simulink library "library_mtu_simulink"  (R2018a)
settings: Solver=VariableStepAuto  StartTime=0.0  StopTime=10.0  RelTol=1e-3  EnableMultiTasking=on
undefined symbols (not defined in the file or in its folder): AP, MP, PA
settings Model: Creator=danielhaeufle  LastModifiedBy=katrinstollenmaier
settings DataIOCC: LimitDataPoints=on
settings OptimizationCC: LifeSpan=inf
settings DebuggingCC: AllowSymbolicDim=off  SFUnexpectedBacktrackingDiag=warning  SFNoUnconditionalDefaultTransitionDiag=warning  SFExecutionAtInitializationDiag=none
settings ModelReferenceCC: PropagateSignalLabelsOutOfModel=off
settings CodeAppCC: StateflowObjectComments=on
settings GRTTargetCC: TargetLangStandard=C89/C90 (ANSI)
settings ConfigComp: CovMetricSettings=dw  CovHtmlReporting=on  CovSaveCumulativeToWorkspaceVar=on  CovSaveSingleToWorkspaceVar=on  CovExternalEMLEnable=off

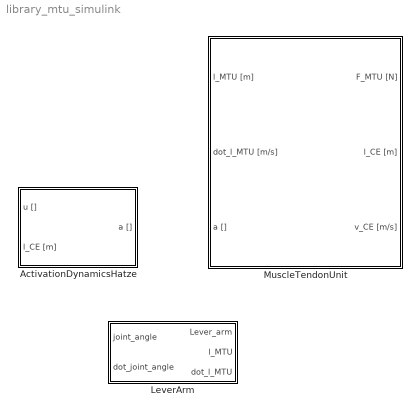
== system library_mtu_simulink ==
  ActivationDynamicsHatze : Subsystem  mask(Activation Dynamics){Act_Param=AP(1), Mus_Param=MP(1)}
      mask prompts: Act_Param "Activation Parameter Struct"; Mus_Param "Muscle Parameter Struct"
      mask help:
      | This block solves the ODE linking neural muscle stimulation u(t) to muscle
      | activity a(t).
      mask Display: %text(.35,.3, 'Aktivierung')
  LeverArm : Subsystem  mask(Lever arm calculations){Lev_Param=PA.Leverxxx}
      mask prompts: Lev_Param "Lever Arm Parameter Struct"
      mask help:
      | This block is the link between joint angles and muscle tendon unit length
      | (l_MTU and dot_l_MTU). In this version, a constant lever arm model is
      | implemented.
  MuscleTendonUnit : Subsystem  mask(Muscle Tendon Complex Model){Mus_Param=MP(1)}
      mask prompts: Mus_Param "Muscle parameter struct"
      mask help: This block returns the muscle tendon complex (MTC) force based on muscle length l_MTC, contraction velocity dot_l_MTC, and activity q
      mask Help:
      | Copyright (c) 2013, D. Haeufle, M. Guenther, A. Bayer, and S. Schmitt
      | All rights reserved.
      | 
      | Redistribution and use in source and binary forms, with or without modification, are permitted provided that the following conditions are met:
      | 
      |     Redistributions of source code must retain the above copyright notice, this list of conditions and the following disclaimer.
      |     Redistributions in binary form must reproduce the above copyright notice, this list of conditions and the following disclaimer in the documentation and/or other materials provided with the distribution.
      |     Neither the name of the <ORGANIZATION> nor the names of its contributors may be used to endorse or promote products derived from this software without specific prior written permission.
      | 
      | THIS SOFTWARE IS PROVIDED BY THE COPYRIGHT HOLDERS AND CONTRIBUTORS "AS IS" AND ANY EXPRESS OR IMPLIED WARRANTIES, INCLUDING, BUT NOT LIMITED TO, THE IMPLIED WARRANTIES OF MERCHANTABILITY AND FITNESS FOR A PARTICULAR PURPOSE ARE DISCLAIMED. IN NO EVENT SHALL THE COPYRIGHT HOLDER OR CONTRIBUTORS BE LIABLE FOR ANY DIRECT, INDIRECT, INCIDENTAL, SPECIAL, EXEMPLARY, OR CONSEQUENTIAL DAMAGES (INCLUDING, BUT NOT LIMITED TO, PROCUREMENT OF SUBSTITUTE GOODS OR SERVICES; LOSS OF USE, DATA, OR PROFITS; OR BUSINESS INTERRUPTION) HOWEVER CAUSED AND ON ANY THEORY OF LIABILITY, WHETHER IN CONTRACT, STRICT LIABILITY, OR TORT (INCLUDING NEGLIGENCE OR OTHERWISE) ARISING IN ANY WAY OUT OF THE USE OF THIS SOFTWARE, EVEN IF ADVISED OF THE POSSIBILITY OF SUCH DAMAGE.
      mask Display: patch([4 4 4 4 3.5 3 2.6 2.2 2 2.2 2.6 3 3.5 4 4 4 4 7 7 7 7 7.5 8 8.4 8.8 9 8.8 8.4 8 7.5 7 7 7 7 4]/20+0.2, [0 2:17 17:-1:2 0 0]/17,[1 0 0])

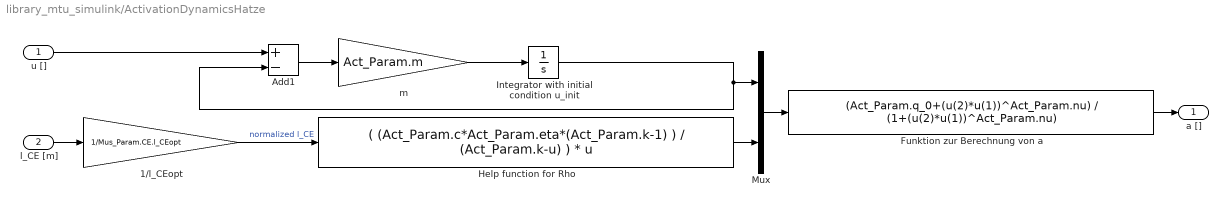
== system library_mtu_simulink/ActivationDynamicsHatze ==
  u [] : Inport
  l_CE [m] : Inport  Port=2
  1/l_CEopt : Gain  Gain=1/Mus_Param.CE.l_CEopt
  Add1 : Sum  Inputs=+-
  Funktion zur Berechnung von a : Fcn  Expr=(Act_Param.q_0+(u(2)*u(1))^Act_Param.nu) / (1+(u(2)*u(1))^Act_Param.nu)
  Help function for Rho : Fcn  Expr=( (Act_Param.c*Act_Param.eta*(Act_Param.k-1) ) / (Act_Param.k-u) ) * u
  Integrator with initial condition u_init : Integrator  InitialCondition=Act_Param.u_init
  Mux : Mux  Inputs=2
  m : Gain  Gain=Act_Param.m
  a [] : Outport
  wires:
  Add1/1 -> m/1
  m/1 -> Integrator with initial condition u_init/1
  Integrator with initial condition u_init/1 -> Add1/2, Mux/1
  Help function for Rho/1 -> Mux/2
  Mux/1 -> Funktion zur Berechnung von a/1
  l_CE [m]/1 -> 1/l_CEopt/1
  Funktion zur Berechnung von a/1 -> a []/1
  u []/1 -> Add1/1
  1/l_CEopt/1 -> Help function for Rho/1  "normalized l_CE"

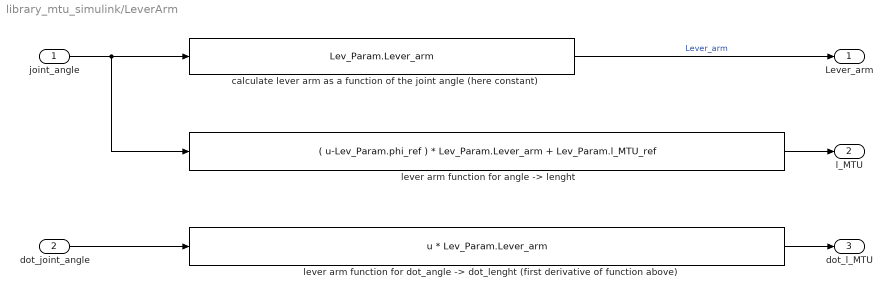
== system library_mtu_simulink/LeverArm ==
  joint_angle : Inport
  dot_joint_angle : Inport  Port=2
  calculate lever arm as a function of the joint angle (here constant) : Fcn  Expr=Lev_Param.Lever_arm
  "lever arm function for angle -> lenght" : Fcn  Expr=( u-Lev_Param.phi_ref ) * Lev_Param.Lever_arm + Lev_Param.l_MTU_ref
  "lever arm function for dot_angle -> dot_lenght (first derivative of function above)" : Fcn  Expr=u * Lev_Param.Lever_arm
  Lever_arm : Outport
  l_MTU : Outport  Port=2
  dot_l_MTU : Outport  Port=3
  wires:
  joint_angle/1 -> calculate lever arm as a function of the joint angle (here constant)/1, "lever arm function for angle -> lenght"/1
  "lever arm function for angle -> lenght"/1 -> l_MTU/1
  "lever arm function for dot_angle -> dot_lenght (first derivative of function above)"/1 -> dot_l_MTU/1
  dot_joint_angle/1 -> "lever arm function for dot_angle -> dot_lenght (first derivative of function above)"/1
  calculate lever arm as a function of the joint angle (here constant)/1 -> Lever_arm/1  "Lever_arm"

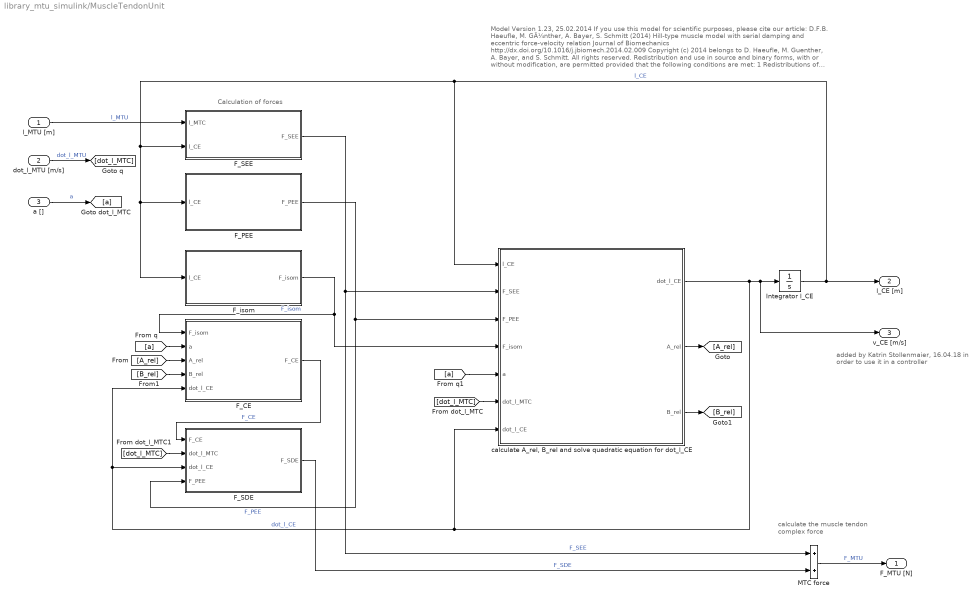
== system library_mtu_simulink/MuscleTendonUnit ==
  note: added by Katrin Stollenmaier,
      | 16.04.18 in order to use it in a controller
  note: Calculation of forces
  note: calculate the
      | muscle tendon complex
      | force
  note: Model Version 1.23, 25.02.2014
      |
      | If you use this model for scientific purposes, please cite our article:
      | D.F.B. Haeufle, M. GÃ¼nther, A. Bayer, S. Schmitt (2014)
      | Hill-type muscle model with serial damping and eccentric force-velocity relation
      | Journal of Biomechanics http://dx.doi.org/10.1016/j.jbiomech.2014.02.009
      |
      |
      | Copyright (c) 2014 belongs to D. Haeufle, M. Guenther, A. Bayer, and S. Schmitt. All rights reserved.
      | Redistribution and use in source and binary forms, with or without modification, are permitted provided that the following conditions are met:
      |
      |  1 Redistributions of source code must retain the above copyright notice,
      |    this list of conditions and the following disclaimer.
      |  2 Redistributions in binary form must reproduce the above copyright
      |    notice, this list of conditions and the following disclaimer in the
      |    documentation and/or other materials provided with the distribution.
      |  3 Neither the name of the owner nor the names of its contributors may be
      |    used to endorse or promote products derived from this software without
      |    specific prior written permission.
      |
      | THIS SOFTWARE IS PROVIDED BY THE COPYRIGHT HOLDERS AND CONTRIBUTORS "AS IS"
      | AND ANY EXPRESS OR IMPLIED WARRANTIES, INCLUDING, BUT NOT LIMITED TO, THE IMPLIED WARRANTIES OF
      | MERCHANTABILITY AND FITNESS FOR A PARTICULAR PURPOSE ARE DISCLAIMED.
      |  IN NO EVENT SHALL THE COPYRIGHT HOLDER BE LIABLE FOR ANY DIRECT, INDIRECT,
      | INCIDENTAL, SPECIAL, EXEMPLARY, OR CONSEQUENTIAL DAMAGES (INCLUDING, BUT
      | NOT LIMITED TO, PROCUREMENT OF SUBSTITUTE GOODS OR SERVICES; LOSS
      | OF USE, DATA, OR PROFITS; OR BUSINESS INTERRUPTION) HOWEVER CAUSED AND ON ANY
      | THEORY OF LIABILITY, WHETHER IN CONTRACT, STRICT LIABILITY, OR TORT (INCLUDING
      | NEGLIGENCE OR OTHERWISE) ARISING IN ANY WAY OUT OF THE USE OF THIS SOFTWARE,
      | EVEN IF ADVISED OF THE POSSIBILITY OF SUCH DAMAGE.
  l_MTU [m] : Inport
  dot_l_MTU [m/s] : Inport  Port=2
  a [] : Inport  Port=3
  F_CE : Subsystem
  F_PEE : Subsystem
  F_SDE : Subsystem
  F_SEE : Subsystem
  F_isom : Subsystem
  Integrator l_CE : Integrator  InitialCondition=Mus_Param.CE.l_CE_init
  MTC force : Sum
  "calculate A_rel, B_rel and solve quadratic equation for dot_l_CE" : Subsystem
  F_MTU [N] : Outport
  l_CE [m] : Outport  Port=2
  "v_CE [m/s] " : Outport  Port=3
  wires:
  F_isom/1(F_isom) -> "calculate A_rel, B_rel and solve quadratic equation for dot_l_CE"/4(F_isom), F_CE/1(F_isom)  "F_isom"
  F_PEE/1(F_PEE) -> F_SDE/4(F_PEE), "calculate A_rel, B_rel and solve quadratic equation for dot_l_CE"/3(F_PEE)  "F_PEE"
  F_SEE/1(F_SEE) -> MTC force/1, "calculate A_rel, B_rel and solve quadratic equation for dot_l_CE"/2(F_SEE)  "F_SEE"
  Integrator l_CE/1 -> l_CE [m]/1, "calculate A_rel, B_rel and solve quadratic equation for dot_l_CE"/1(l_CE), F_SEE/2(l_CE), F_isom/1(l_CE), F_PEE/1(l_CE)  "l_CE"
  F_CE/1(F_CE) -> F_SDE/1(F_CE)  "F_CE"
  F_SDE/1(F_SDE) -> MTC force/2  "F_SDE"
  MTC force/1 -> F_MTU [N]/1  "F_MTU"
  l_MTU [m]/1 -> F_SEE/1(l_MTC)  "l_MTU"
  "calculate A_rel, B_rel and solve quadratic equation for dot_l_CE"/1("dot_l_CE ") -> "calculate A_rel, B_rel and solve quadratic equation for dot_l_CE"/7(dot_l_CE), F_CE/5(dot_l_CE), F_SDE/3(dot_l_CE), "v_CE [m/s] "/1, Integrator l_CE/1  "dot_l_CE"
  [a] -> F_CE/2(a)
  [a] -> "calculate A_rel, B_rel and solve quadratic equation for dot_l_CE"/5("a ")
  [dot_l_MTC] -> "calculate A_rel, B_rel and solve quadratic equation for dot_l_CE"/6(dot_l_MTC)
  [dot_l_MTC] -> F_SDE/2(dot_l_MTC)
  "calculate A_rel, B_rel and solve quadratic equation for dot_l_CE"/2(A_rel) -> [A_rel]
  "calculate A_rel, B_rel and solve quadratic equation for dot_l_CE"/3(B_rel) -> [B_rel]
  [A_rel] -> F_CE/3(A_rel)
  [B_rel] -> F_CE/4(B_rel)
  dot_l_MTU [m/s]/1 -> [dot_l_MTC]  "dot_l_MTU"
  a []/1 -> [a]  "a"

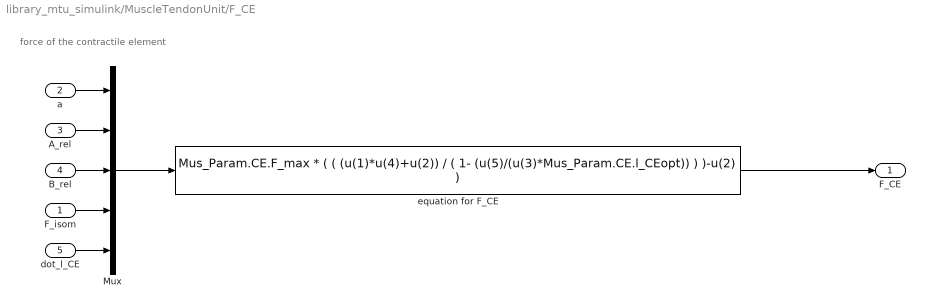
== system library_mtu_simulink/MuscleTendonUnit/F_CE ==
  note: force of the contractile element
  F_isom : Inport
  a : Inport  Port=2
  A_rel : Inport  Port=3
  B_rel : Inport  Port=4
  dot_l_CE : Inport  Port=5
  Mux : Mux  Inputs=5
  equation for F_CE : Fcn  Expr="Mus_Param.CE.F_max * (  ( (u(1)*u(4)+u(2)) / ( 1- (u(5)/(u(3)*Mus_Param.CE.l_CEopt)) ) )-u(2) )"
  F_CE : Outport
  wires:
  Mux/1 -> equation for F_CE/1
  a/1 -> Mux/1
  A_rel/1 -> Mux/2
  B_rel/1 -> Mux/3
  F_isom/1 -> Mux/4
  dot_l_CE/1 -> Mux/5
  equation for F_CE/1 -> F_CE/1

== system library_mtu_simulink/MuscleTendonUnit/F_PEE ==
  note: Parallel elastic element force
      |
      | is only calculated if l_CE>PEE slack length
      | to avoid complex numbers with
      | non-integer exponents
  l_CE : Inport
  "F_PEE " : Subsystem
  l_PEE > slack length? : Fcn  Expr=(u>=Mus_Param.PEE.l_PEE0)
  F_PEE : Outport
  wires:
  l_CE/1 -> l_PEE > slack length?/1, "F_PEE "/1(l_PEE)
  "F_PEE "/1(Out1) -> F_PEE/1
  l_PEE > slack length?/1 -> "F_PEE "/Enable

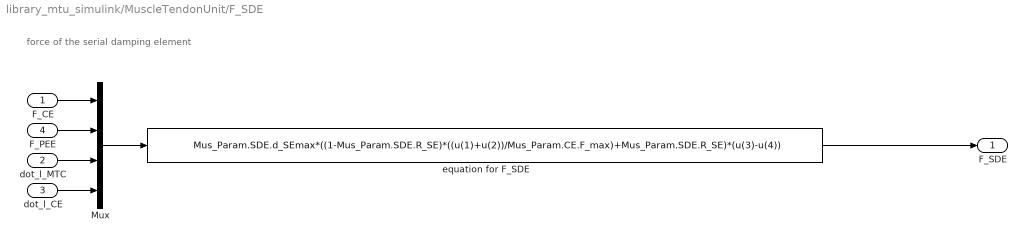
== system library_mtu_simulink/MuscleTendonUnit/F_SDE ==
  note: force of the serial damping element
  F_CE : Inport
  dot_l_MTC : Inport  Port=2
  dot_l_CE : Inport  Port=3
  F_PEE : Inport  Port=4
  Mux : Mux
  equation for F_SDE : Fcn  Expr=Mus_Param.SDE.d_SEmax*((1-Mus_Param.SDE.R_SE)*((u(1)+u(2))/Mus_Param.CE.F_max)+Mus_Param.SDE.R_SE)*(u(3)-u(4))
  F_SDE : Outport
  wires:
  Mux/1 -> equation for F_SDE/1
  F_PEE/1 -> Mux/2
  F_CE/1 -> Mux/1
  equation for F_SDE/1 -> F_SDE/1
  dot_l_MTC/1 -> Mux/3
  dot_l_CE/1 -> Mux/4

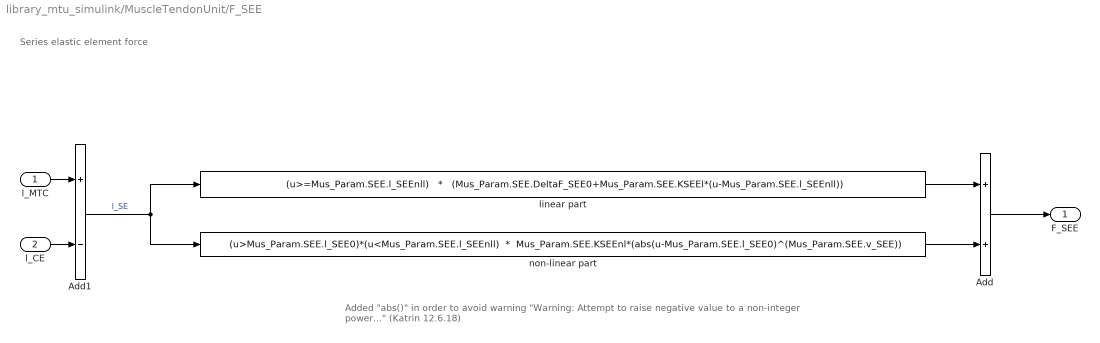
== system library_mtu_simulink/MuscleTendonUnit/F_SEE ==
  note: Added "abs()" in order to avoid warning "Warning: Attempt to raise negative value to a non-integer power..."
      | (Katrin 12.6.18)
  note: Series elastic element force
  l_MTC : Inport
  l_CE : Inport  Port=2
  Add : Sum
  Add1 : Sum  Inputs=+-
  linear part : Fcn  Expr="(u>=Mus_Param.SEE.l_SEEnll)   *   (Mus_Param.SEE.DeltaF_SEE0+Mus_Param.SEE.KSEEl*(u-Mus_Param.SEE.l_SEEnll))"
  non-linear part : Fcn  Expr="(u>Mus_Param.SEE.l_SEE0)*(u<Mus_Param.SEE.l_SEEnll)  *  Mus_Param.SEE.KSEEnl*(abs(u-Mus_Param.SEE.l_SEE0)^(Mus_Param.SEE.v_SEE))"
  F_SEE : Outport
  wires:
  linear part/1 -> Add/1
  Add1/1 -> linear part/1, non-linear part/1  "l_SE"
  l_MTC/1 -> Add1/1
  Add/1 -> F_SEE/1
  l_CE/1 -> Add1/2
  non-linear part/1 -> Add/2

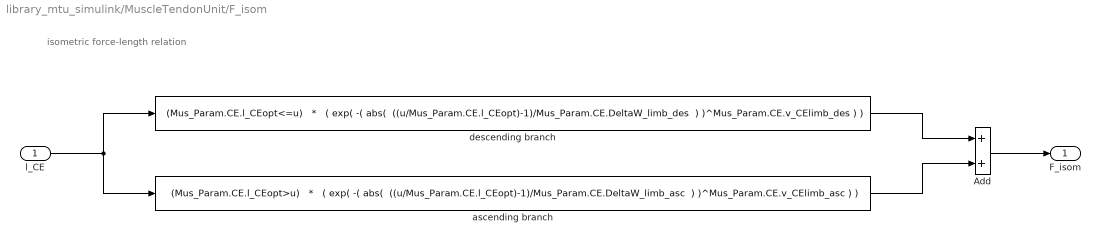
== system library_mtu_simulink/MuscleTendonUnit/F_isom ==
  note: isometric force-length relation
  l_CE : Inport
  Add : Sum
  ascending branch : Fcn  Expr="(Mus_Param.CE.l_CEopt>u)   *   ( exp( -( abs(  ((u/Mus_Param.CE.l_CEopt)-1)/Mus_Param.CE.DeltaW_limb_asc  ) )^Mus_Param.CE.v_CElimb_asc ) )"
  descending branch : Fcn  Expr="(Mus_Param.CE.l_CEopt<=u)   *   ( exp( -( abs(  ((u/Mus_Param.CE.l_CEopt)-1)/Mus_Param.CE.DeltaW_limb_des  ) )^Mus_Param.CE.v_CElimb_des ) )"
  F_isom : Outport
  wires:
  descending branch/1 -> Add/1
  ascending branch/1 -> Add/2
  Add/1 -> F_isom/1
  l_CE/1 -> descending branch/1, ascending branch/1

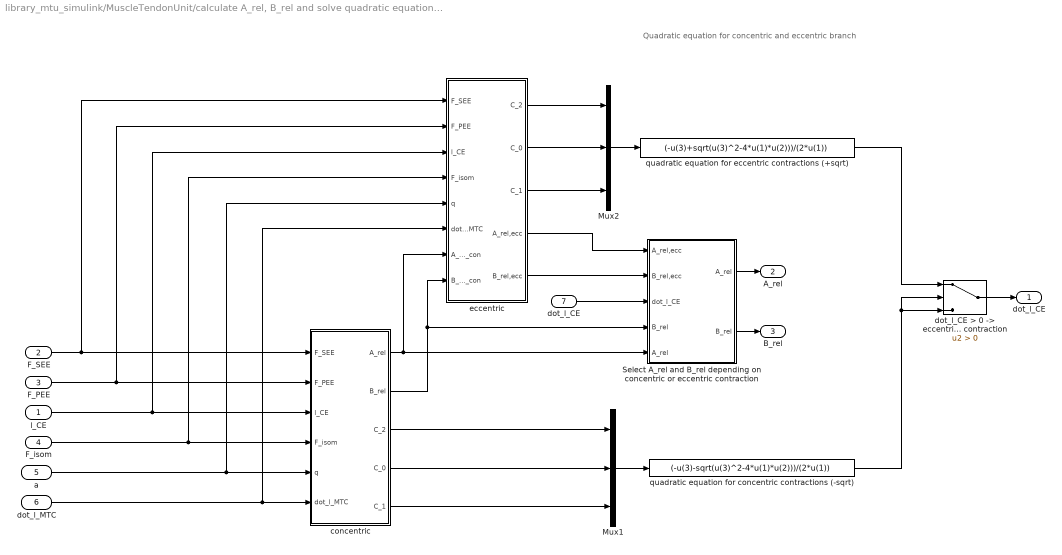
== system library_mtu_simulink/MuscleTendonUnit/calculate A_rel, B_rel and solve quadratic equation for dot_l_CE ==
  note: Quadratic equation for concentric and eccentric branch
  l_CE : Inport
  F_SEE : Inport  Port=2
  F_PEE : Inport  Port=3
  F_isom : Inport  Port=4
  "a " : Inport  Port=5
  dot_l_MTC : Inport  Port=6
  dot_l_CE : Inport  Port=7
  Mux1 : Mux  Inputs=3
  Mux2 : Mux  Inputs=3
  Select A_rel and B_rel depending on concentric or eccentric contraction : Subsystem
  concentric : Subsystem
  "dot_l_CE > 0 -> eccentric contraction" : Switch  Criteria=u2 > Threshold  ZeroCross=off
  eccentric : Subsystem
  quadratic equation for concentric contractions (-sqrt) : Fcn  Expr=(-u(3)-sqrt(u(3)^2-4*u(1)*u(2)))/(2*u(1))
  quadratic equation for eccentric contractions (+sqrt) : Fcn  Expr=(-u(3)+sqrt(u(3)^2-4*u(1)*u(2)))/(2*u(1))
  "dot_l_CE " : Outport
  A_rel : Outport  Port=2
  B_rel : Outport  Port=3
  wires:
  dot_l_MTC/1 -> eccentric/6(dot_l_MTC), concentric/6(dot_l_MTC)
  F_PEE/1 -> eccentric/2(F_PEE), concentric/2(F_PEE)
  l_CE/1 -> eccentric/3(l_CE), concentric/3(l_CE)
  concentric/2(B_rel) -> eccentric/8(B_rel_con), Select A_rel and B_rel depending on concentric or eccentric contraction/4(B_rel)
  F_SEE/1 -> eccentric/1(F_SEE), concentric/1(F_SEE)
  F_isom/1 -> eccentric/4(F_isom), concentric/4(F_isom)
  "a "/1 -> eccentric/5(q), concentric/5(q)
  concentric/1(A_rel) -> eccentric/7(A_rel_con), Select A_rel and B_rel depending on concentric or eccentric contraction/5(A_rel)
  "dot_l_CE > 0 -> eccentric contraction"/1 -> "dot_l_CE "/1
  concentric/3("C_2 ") -> Mux1/1
  concentric/4("C_0 ") -> Mux1/2
  concentric/5("C_1 ") -> Mux1/3
  Mux1/1 -> quadratic equation for concentric contractions (-sqrt)/1
  quadratic equation for concentric contractions (-sqrt)/1 -> "dot_l_CE > 0 -> eccentric contraction"/2, "dot_l_CE > 0 -> eccentric contraction"/3
  quadratic equation for eccentric contractions (+sqrt)/1 -> "dot_l_CE > 0 -> eccentric contraction"/1
  Mux2/1 -> quadratic equation for eccentric contractions (+sqrt)/1
  eccentric/1(C_2) -> Mux2/1
  eccentric/2(C_0) -> Mux2/2
  eccentric/3(C_1) -> Mux2/3
  eccentric/4(A_rel,ecc) -> Select A_rel and B_rel depending on concentric or eccentric contraction/1(A_rel,ecc)
  eccentric/5(B_rel,ecc) -> Select A_rel and B_rel depending on concentric or eccentric contraction/2(B_rel,ecc)
  dot_l_CE/1 -> Select A_rel and B_rel depending on concentric or eccentric contraction/3(dot_l_CE)
  Select A_rel and B_rel depending on concentric or eccentric contraction/1(" A_rel") -> A_rel/1
  Select A_rel and B_rel depending on concentric or eccentric contraction/2("B_rel ") -> B_rel/1

== system library_mtu_simulink/MuscleTendonUnit/F_PEE/F_PEE  ==
  note: Added "abs()" in order to avoid warning "Warning: Attempt to raise negative value to a non-integer power..."
      | (Katrin 12.6.18)
  l_PEE : Inport
  Enable : EnablePort  StatesWhenEnabling=reset
  "F_PEE " : Fcn  Expr=Mus_Param.PEE.K_PEE*abs(u-Mus_Param.PEE.l_PEE0)^(Mus_Param.PEE.v_PEE)
  Out1 : Outport  InitialOutput=0
  wires:
  l_PEE/1 -> "F_PEE "/1
  "F_PEE "/1 -> Out1/1

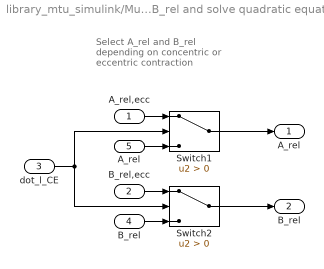
== system library_mtu_simulink/MuscleTendonUnit/calculate A_rel, B_rel and solve quadratic equation for dot_l_CE/Select A_rel and B_rel depending on concentric or eccentric contraction ==
  note: Select A_rel and B_rel
      | depending on concentric or
      | eccentric contraction
  A_rel,ecc : Inport
  B_rel,ecc : Inport  Port=2
  dot_l_CE : Inport  Port=3
  B_rel : Inport  Port=4
  A_rel : Inport  Port=5
  Switch1 : Switch  Criteria=u2 > Threshold  ZeroCross=off
  Switch2 : Switch  Criteria=u2 > Threshold  ZeroCross=off
  " A_rel" : Outport
  "B_rel " : Outport  Port=2
  wires:
  dot_l_CE/1 -> Switch1/2, Switch2/2
  Switch1/1 -> " A_rel"/1
  Switch2/1 -> "B_rel "/1
  A_rel,ecc/1 -> Switch1/1
  B_rel,ecc/1 -> Switch2/1
  A_rel/1 -> Switch1/3
  B_rel/1 -> Switch2/3

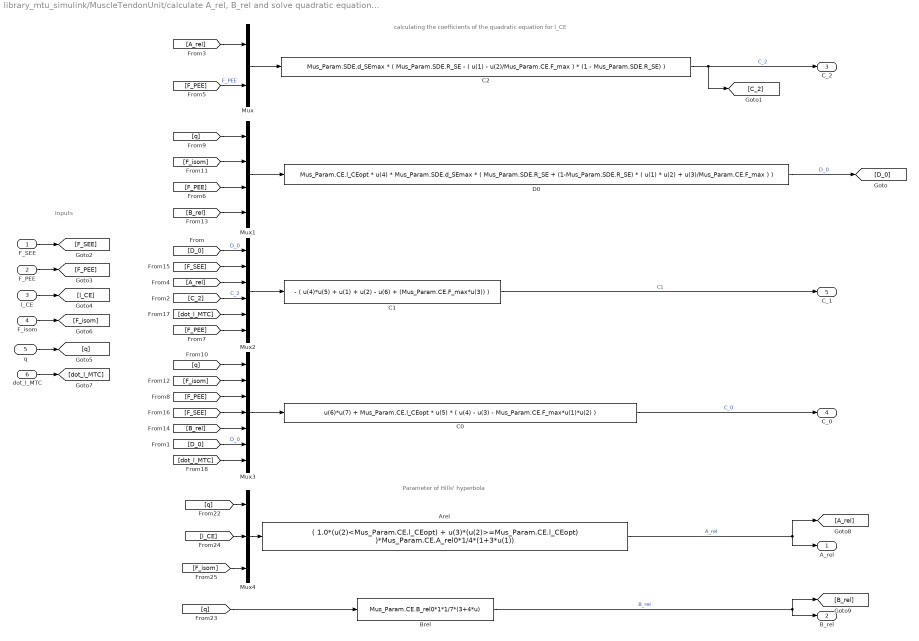
== system library_mtu_simulink/MuscleTendonUnit/calculate A_rel, B_rel and solve quadratic equation for dot_l_CE/concentric ==
  note: Inputs
  note: calculating the coefficients of the quadratic equation for l_CE
  note: Parameter of Hills' hyperbola
  F_SEE : Inport
  F_PEE : Inport  Port=2
  l_CE : Inport  Port=3
  F_isom : Inport  Port=4
  q : Inport  Port=5
  dot_l_MTC : Inport  Port=6
  Arel : Fcn  Expr=( 1.0*(u(2)<Mus_Param.CE.l_CEopt) + u(3)*(u(2)>=Mus_Param.CE.l_CEopt) )*Mus_Param.CE.A_rel0*1/4*(1+3*u(1))
  Brel : Fcn  Expr=Mus_Param.CE.B_rel0*1*1/7*(3+4*u)
  C0 : Fcn  Expr=u(6)*u(7) + Mus_Param.CE.l_CEopt * u(5) * ( u(4) - u(3) - Mus_Param.CE.F_max*u(1)*u(2) )
  C1 : Fcn  Expr=- ( u(4)*u(5) + u(1) + u(2) - u(6) + (Mus_Param.CE.F_max*u(3)) )
  C2 : Fcn  Expr=Mus_Param.SDE.d_SEmax * ( Mus_Param.SDE.R_SE - ( u(1) - u(2)/Mus_Param.CE.F_max ) * (1 - Mus_Param.SDE.R_SE) )
  "D0 " : Fcn  Expr=Mus_Param.CE.l_CEopt * u(4) * Mus_Param.SDE.d_SEmax * ( Mus_Param.SDE.R_SE + (1-Mus_Param.SDE.R_SE) * ( u(1) * u(2) + u(3)/Mus_Param.CE.F_max ) )
  Mux : Mux  Inputs=2
  Mux1 : Mux
  Mux2 : Mux  Inputs=6
  Mux3 : Mux  Inputs=7
  Mux4 : Mux  Inputs=3
  A_rel : Outport
  B_rel : Outport  Port=2
  "C_2 " : Outport  Port=3
  "C_0 " : Outport  Port=4
  "C_1 " : Outport  Port=5
  wires:
  Arel/1 -> A_rel/1, [A_rel]  "A_rel"
  dot_l_MTC/1 -> [dot_l_MTC]
  Brel/1 -> [B_rel], B_rel/1  "B_rel"
  Mux/1 -> C2/1
  C2/1 -> "C_2 "/1, [C_2]  "C_2"
  Mux1/1 -> "D0 "/1
  "D0 "/1 -> [D_0]  "D_0"
  Mux2/1 -> C1/1
  [D_0] -> Mux2/1  "D_0"
  [C_2] -> Mux2/4  "C_2"
  C1/1 -> "C_1 "/1  "C1"
  Mux3/1 -> C0/1
  [D_0] -> Mux3/6  "D_0"
  C0/1 -> "C_0 "/1  "C_0"
  [A_rel] -> Mux/1
  F_SEE/1 -> [F_SEE]
  F_PEE/1 -> [F_PEE]
  l_CE/1 -> [l_CE]
  q/1 -> [q]
  F_isom/1 -> [F_isom]
  [A_rel] -> Mux2/3
  [dot_l_MTC] -> Mux3/7
  [F_PEE] -> Mux/2  "F_PEE"
  [q] -> Mux1/1
  [F_isom] -> Mux1/2
  [F_PEE] -> Mux1/3
  [B_rel] -> Mux1/4
  [F_SEE] -> Mux2/2
  [dot_l_MTC] -> Mux2/5
  [F_PEE] -> Mux2/6
  [q] -> Mux3/1
  [F_isom] -> Mux3/2
  [F_PEE] -> Mux3/3
  [F_SEE] -> Mux3/4
  [B_rel] -> Mux3/5
  Mux4/1 -> Arel/1
  [F_isom] -> Mux4/3
  [l_CE] -> Mux4/2
  [q] -> Mux4/1
  [q] -> Brel/1

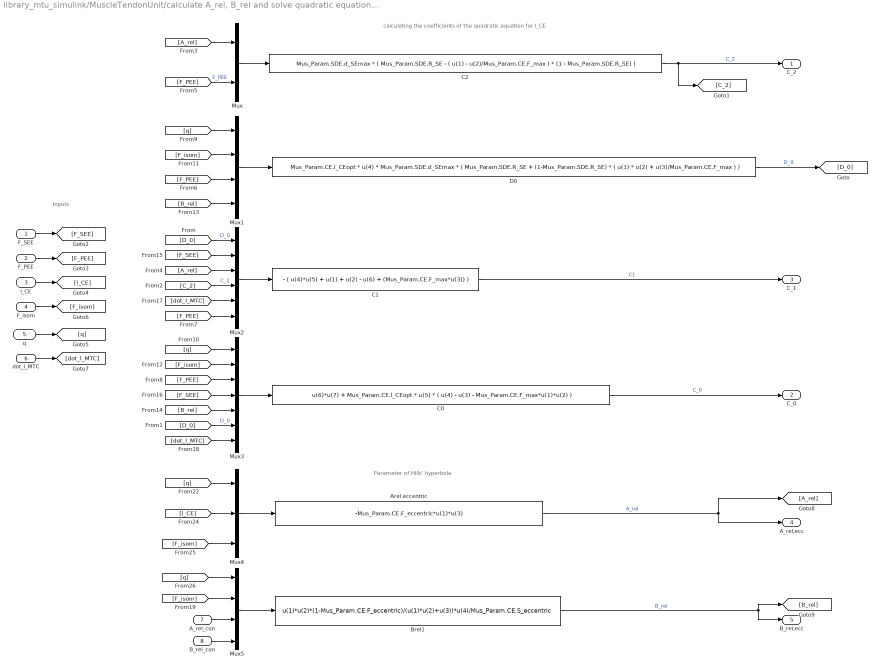
== system library_mtu_simulink/MuscleTendonUnit/calculate A_rel, B_rel and solve quadratic equation for dot_l_CE/eccentric ==
  note: Inputs
  note: calculating the coefficients of the quadratic equation for l_CE
  note: Parameter of Hills' hyperbola
  F_SEE : Inport
  F_PEE : Inport  Port=2
  l_CE : Inport  Port=3
  F_isom : Inport  Port=4
  q : Inport  Port=5
  dot_l_MTC : Inport  Port=6
  A_rel_con : Inport  Port=7
  B_rel_con : Inport  Port=8
  Arel eccentric : Fcn  Expr=-Mus_Param.CE.F_eccentric*u(1)*u(3)
  Brel1 : Fcn  Expr=u(1)*u(2)*(1-Mus_Param.CE.F_eccentric)/(u(1)*u(2)+u(3))*u(4)/Mus_Param.CE.S_eccentric
  C0 : Fcn  Expr=u(6)*u(7) + Mus_Param.CE.l_CEopt * u(5) * ( u(4) - u(3) - Mus_Param.CE.F_max*u(1)*u(2) )
  C1 : Fcn  Expr=- ( u(4)*u(5) + u(1) + u(2) - u(6) + (Mus_Param.CE.F_max*u(3)) )
  C2 : Fcn  Expr=Mus_Param.SDE.d_SEmax * ( Mus_Param.SDE.R_SE - ( u(1) - u(2)/Mus_Param.CE.F_max ) * (1 - Mus_Param.SDE.R_SE) )
  "D0 " : Fcn  Expr=Mus_Param.CE.l_CEopt * u(4) * Mus_Param.SDE.d_SEmax * ( Mus_Param.SDE.R_SE + (1-Mus_Param.SDE.R_SE) * ( u(1) * u(2) + u(3)/Mus_Param.CE.F_max ) )
  Mux : Mux  Inputs=2
  Mux1 : Mux
  Mux2 : Mux  Inputs=6
  Mux3 : Mux  Inputs=7
  Mux4 : Mux  Inputs=3
  Mux5 : Mux
  C_2 : Outport
  C_0 : Outport  Port=2
  C_1 : Outport  Port=3
  A_rel,ecc : Outport  Port=4
  B_rel,ecc : Outport  Port=5
  wires:
  Arel eccentric/1 -> A_rel,ecc/1, [A_rel]  "A_rel"
  dot_l_MTC/1 -> [dot_l_MTC]
  Brel1/1 -> [B_rel], B_rel,ecc/1  "B_rel"
  Mux/1 -> C2/1
  C2/1 -> C_2/1, [C_2]  "C_2"
  Mux1/1 -> "D0 "/1
  "D0 "/1 -> [D_0]  "D_0"
  Mux2/1 -> C1/1
  [D_0] -> Mux2/1  "D_0"
  [C_2] -> Mux2/4  "C_2"
  C1/1 -> C_1/1  "C1"
  Mux3/1 -> C0/1
  [D_0] -> Mux3/6  "D_0"
  C0/1 -> C_0/1  "C_0"
  [A_rel] -> Mux/1
  F_SEE/1 -> [F_SEE]
  F_PEE/1 -> [F_PEE]
  l_CE/1 -> [l_CE]
  q/1 -> [q]
  F_isom/1 -> [F_isom]
  [A_rel] -> Mux2/3
  [dot_l_MTC] -> Mux3/7
  [F_PEE] -> Mux/2  "F_PEE"
  [q] -> Mux1/1
  [F_isom] -> Mux1/2
  [F_PEE] -> Mux1/3
  [B_rel] -> Mux1/4
  [F_SEE] -> Mux2/2
  [dot_l_MTC] -> Mux2/5
  [F_PEE] -> Mux2/6
  [q] -> Mux3/1
  [F_isom] -> Mux3/2
  [F_PEE] -> Mux3/3
  [F_SEE] -> Mux3/4
  [B_rel] -> Mux3/5
  Mux4/1 -> Arel eccentric/1
  [F_isom] -> Mux4/3
  [l_CE] -> Mux4/2
  [q] -> Mux4/1
  [q] -> Mux5/1
  [F_isom] -> Mux5/2
  A_rel_con/1 -> Mux5/3
  B_rel_con/1 -> Mux5/4
  Mux5/1 -> Brel1/1
